simulink model "Correccion_Sist_Fisico_MA"  (R2021a)
settings: Solver=VariableStepAuto  StartTime=0.0  StopTime=inf  RelTol=1e-3
values from neighbouring files (symbols this model uses):
  b_cx = 1*10^6    (= 1000000)    [parametros.m]
  b_cy = 1*10^7    (= 10000000)    [parametros.m]
  b_eq = (b_td+b_tm*(r_t^2))/r_td    (= 10803.6)    [parametros.m]
  b_eqh = 2*(b_hd+b_hm*(r_h^2))/r_hd    (= 23253.3333333)    [parametros.m]
  b_ha = b_eqh/r_h - n_h*w_posh*(J_eqh + 0.5*m_l_*r_hd)/r_h    [parametros.m]
  b_hb = 1*10^8    (= 100000000)    [parametros.m]
  b_hEb = 2.2*10^9    (= 2200000000)    [parametros.m]
  b_t = 90    [parametros.m]
  b_ta = n_t*w_post*(r_td*J_eqt/r_t) - r_td*b_eqt/r_t    [parametros.m]
  b_tb = 5*10^6    (= 5000000)    [parametros.m]
  b_tw = 3*10^3    (= 3000)    [parametros.m]
  b_wu = 150    [parametros.m]
  dt = 5e-3    (= 0.005)    [parametros.m]
  g = 9.80665    [parametros.m]
  H_c = 2.5    [parametros.m]
  J_eq = (J_td+J_tm_tb*(r_t^2))/r_td    (= 15000)    [parametros.m]
  J_eqh = 2*(J_hd_hEb+J_hm_hb*(r_h^2))/r_hd    (= 48853.3333333)    [parametros.m]
  K_cy = 1.8*10^9    (= 1800000000)    [parametros.m]
  K_hsa = -n_h*(w_posh^2)*(J_eqh + 0.5*m_l_*r_hd)/r_t    [parametros.m]
  K_hsia = -(w_posh^3)*(J_eqh + 0.5*m_l_*r_hd)/r_t    [parametros.m]
  K_tsa = n_t*(w_post^2)*J_eqt*r_td/r_t    [parametros.m]
  K_tsia = (w_post^3)*J_eqt*r_td/r_t    [parametros.m]
  K_tw = 4.8*10^5    (= 480000)    [parametros.m]
  k_wu = 2.36*10^8    (= 236000000)    [parametros.m]
  lh_inicial = 45-yl_inicial    (= 30)    [parametros.m]
  M_c_MAX = 50000 + M_s    (= 65000)    [parametros.m]
  M_real = 10000    [parametros.m]
  M_s = 15000    [parametros.m]
  M_t = 30000    [parametros.m]
  r_h = 22    [parametros.m]
  r_hd = 0.75    [parametros.m]
  r_t = 30    [parametros.m]
  r_td = 0.5    [parametros.m]
  T_hb_MAX = 5*10^5    (= 500000)    [parametros.m]
  T_hEb_MAX = 1.1*10^6    (= 1100000)    [parametros.m]
  T_hm_MAX = 2*10^5    (= 200000)    [parametros.m]
  T_s2 = 5e-3    (= 0.005)    [parametros.m]
  T_tb_MAX = 5*10^4    (= 50000)    [parametros.m]
  T_tm_MAX = 3*10^4    (= 30000)    [parametros.m]
  tau_hm = 1e-3    (= 0.001)    [parametros.m]
  tau_tm = 1e-3    (= 0.001)    [parametros.m]
  TensionMinima = (M_s*g/2)*0.7    (= 51484.9125)    [parametros.m]
  v_h_MAX_c = +1.5    (= 1.5)    [parametros.m]
  v_t_MAX = +4    (= 4)    [parametros.m]
  v_t_MIN = -4    [parametros.m]
  w_hm_min = pi/4    (= 0.785398163397)    [parametros.m]
  w_tm_min = pi/4    (= 0.785398163397)    [parametros.m]
  xt_inicial = -10    [parametros.m]
  Y_t0 = 45    [parametros.m]
  yl_inicial = 15    [parametros.m]
undefined symbols (not defined in the file or in its folder): DiscIntNeverNeededParam
libraries: simulink x10, dspstat3 x1, vrlib x1
(part 3 of 3)

== stateflow chart Correccion_Sist_Fisico_MA/Chart ==
  note: ---> FINES DE CARRERA:
      |
      | 1. FIN DE CARRERA CARRO:
  state Nivel_1_Apagado
  note: ---> Si el Nivel 1 se encuentra apagodo deberia actuar el Nivel 0
  note: ---> Activado = Freno Energizado = Freno ABIERTO
  note: ---> Desactivado = Freno NO Energizado = Freno CERRADO
  state Nivel_1_Encendido
    state Sobrevelocidad [parallel]
      settings: executionOrder=11
      state CARRO [parallel]
        settings: executionOrder=2
        state Actualizacion_Vel_CARRO
          during:
          dx_t_SobreV = dx_t_ref_man;
        state Analisis_Sobrevelocidad
          entry:
          if (dx_t_ref_man>0)
          dx_t_SobreV = v_t_MAX;
          else
          dx_t_SobreV = v_t_MIN;
          end
        (default) -> Actualizacion_Vel_CARRO
        Actualizacion_Vel_CARRO -> Analisis_Sobrevelocidad : [abs(dx_t_ref_man) > v_t_MAX]
        Analisis_Sobrevelocidad -> Actualizacion_Vel_CARRO : [abs(dx_t_ref_man) <= v_t_MAX]
      state IZAJE [parallel]
        settings: executionOrder=1
        state Actualizacion_Vel_IZAJE
          during:
          dl_h_SobreV = dl_h_ref_man;
        state Analisis_Sobrevelocidad_Pos
          entry:
          dl_h_SobreV = v_h_MAXMIN;
        state Analisis_Sobrevelocidad_Neg
          entry:
          dl_h_SobreV = -v_h_MAXMIN;
        state BAJAR
          entry:
          dl_h_SobreV = v_h_MAX_c*0.1;
        (default) -> Actualizacion_Vel_IZAJE
        Actualizacion_Vel_IZAJE -> Analisis_Sobrevelocidad_Pos [order 1] : [(dl_h_ref_man > v_h_MAXMIN)  && ~sobrecarga ]
        Analisis_Sobrevelocidad_Pos -> Actualizacion_Vel_IZAJE : [(dl_h_ref_man <= v_h_MAXMIN) || sobrecarga ]
        Actualizacion_Vel_IZAJE -> Analisis_Sobrevelocidad_Neg [order 3] : [(dl_h_ref_man < -v_h_MAXMIN)   && ~sobrecarga ]
        Analisis_Sobrevelocidad_Neg -> Actualizacion_Vel_IZAJE : [(dl_h_ref_man >= -v_h_MAXMIN)  || sobrecarga ]
        Actualizacion_Vel_IZAJE -> BAJAR [order 2] : [sobrecarga]
        BAJAR -> Actualizacion_Vel_IZAJE : [~sobrecarga]
    state Fines_de_Carrera [parallel]
      settings: executionOrder=2
      state FIN_DE_CARRERA_CARRO [parallel]
        settings: executionOrder=1
        state Frenar
          entry:
          Detener_CarroFDC = 1;
        state MOVER_CARRO
          during:
          Detener_CarroFDC = 0;
        state No_Frenar
          entry:
          Detener_CarroFDC = 0;
        (default) -> Nivel_1_Encendido.Fines_de_Carrera.FIN_DE_CARRERA_CARRO.No_Frenar
        Nivel_1_Encendido.Fines_de_Carrera.FIN_DE_CARRERA_CARRO.Frenar -> Nivel_1_Encendido.Fines_de_Carrera.FIN_DE_CARRERA_CARRO.MOVER_CARRO [order 2] : [((dx_t_ref_man < 0 && Fin_Der_n) || (dx_t_ref_man > 0 && Fin_Izq_n))]
        Nivel_1_Encendido.Fines_de_Carrera.FIN_DE_CARRERA_CARRO.No_Frenar -> Nivel_1_Encendido.Fines_de_Carrera.FIN_DE_CARRERA_CARRO.Frenar : [Fin_Der_n || Fin_Izq_n]
        Nivel_1_Encendido.Fines_de_Carrera.FIN_DE_CARRERA_CARRO.MOVER_CARRO -> Nivel_1_Encendido.Fines_de_Carrera.FIN_DE_CARRERA_CARRO.Frenar : [(dx_t_ref_man >= 0 && Fin_Der_n) || (dx_t_ref_man <= 0 && Fin_Izq_n) || (~Fin_Der_n && ~Fin_Izq_n) ]
        Nivel_1_Encendido.Fines_de_Carrera.FIN_DE_CARRERA_CARRO.Frenar -> Nivel_1_Encendido.Fines_de_Carrera.FIN_DE_CARRERA_CARRO.No_Frenar [order 1] : [~Fin_Der_n && ~Fin_Izq_n]
      state FIN_DE_CARRERA_IZAJE [parallel]
        settings: executionOrder=2
        state Frenar
          entry:
          Detener_IzajeFDC = 1;
        state MOVER_IZAJE
          during:
          Detener_IzajeFDC = 0;
        state No_Frenar
          entry:
          Detener_IzajeFDC = 0;
        (default) -> Nivel_1_Encendido.Fines_de_Carrera.FIN_DE_CARRERA_IZAJE.No_Frenar
        Nivel_1_Encendido.Fines_de_Carrera.FIN_DE_CARRERA_IZAJE.Frenar -> Nivel_1_Encendido.Fines_de_Carrera.FIN_DE_CARRERA_IZAJE.MOVER_IZAJE [order 2] : [((dl_h_ref_man > 0 && Fin_Sup_n) || (dl_h_ref_man < 0 && Fin_Inf_n))]
        Nivel_1_Encendido.Fines_de_Carrera.FIN_DE_CARRERA_IZAJE.No_Frenar -> Nivel_1_Encendido.Fines_de_Carrera.FIN_DE_CARRERA_IZAJE.Frenar : [Fin_Sup_n || Fin_Inf_n]
        Nivel_1_Encendido.Fines_de_Carrera.FIN_DE_CARRERA_IZAJE.MOVER_IZAJE -> Nivel_1_Encendido.Fines_de_Carrera.FIN_DE_CARRERA_IZAJE.Frenar : [(dl_h_ref_man <= 0 && Fin_Sup_n) || (dl_h_ref_man >= 0 && Fin_Inf_n) || (~Fin_Sup_n && ~Fin_Inf_n) ]
        Nivel_1_Encendido.Fines_de_Carrera.FIN_DE_CARRERA_IZAJE.Frenar -> Nivel_1_Encendido.Fines_de_Carrera.FIN_DE_CARRERA_IZAJE.No_Frenar [order 1] : [~Fin_Sup_n && ~Fin_Inf_n]
    state Frenos [parallel]
      settings: executionOrder=4
      note: % Freno desactivado = Frenando
      state FRENO_CARRO [parallel]
        settings: executionOrder=1
        state No_Frenando
          entry:
          BRK_t = 1;
          Detener_CarroFR = 0;
        state Frenando
          entry:
          BRK_t = 0;
          Detener_CarroFR = 1;
        (default) -> Nivel_1_Encendido.Frenos.FRENO_CARRO.Frenando
        Nivel_1_Encendido.Frenos.FRENO_CARRO.No_Frenando -> Nivel_1_Encendido.Frenos.FRENO_CARRO.Frenando : [(abs(w_tm) < w_tm_min && Freno_Carro_Man) || (Emergencia == 2 && ~Salida_E_C) || sobrecarga || ( dx_t_ref == 0 && dx_t_SobreV == 0) ||  Detener_CarroFDC || (dx_t_ref * dx_t_ref_man < 0) ]
        Nivel_1_Encendido.Frenos.FRENO_CARRO.Frenando -> Nivel_1_Encendido.Frenos.FRENO_CARRO.No_Frenando : [Tmt_disp && ~Freno_Carro_Man && (Emergencia == 0 || Salida_E_C) && ~sobrecarga && ( dx_t_ref ~= 0 || dx_t_SobreV ~= 0) && ~Detener_CarroFDC && (dx_t_ref * dx_t_ref_man >= 0)]
      state FRENO_IZAJE [parallel]
        settings: executionOrder=2
        state No_Frenando
          entry:
          BRK_h = 1;
          Detener_IzajeFR = 0;
        state Frenando
          entry:
          BRK_h = 0;
          Detener_IzajeFR = 1;
        (default) -> Nivel_1_Encendido.Frenos.FRENO_IZAJE.Frenando
        Nivel_1_Encendido.Frenos.FRENO_IZAJE.No_Frenando -> Nivel_1_Encendido.Frenos.FRENO_IZAJE.Frenando : [(abs(w_hm) < w_hm_min && Freno_Izaje_Man) || (Emergencia == 3 && ~Salida_E_I)  || (sobrecarga && dl_h_ref <= 0) || ( dl_h_ref == 0 && dl_h_SobreV == 0) || Detener_IzajeFDC || ~Cable_Tenso || (45-l_h < y_obstaculo-0.15 && dl_h_ref_man >= 0) || (dl_h_ref * dl_h_ref_man < 0)]
        Nivel_1_Encendido.Frenos.FRENO_IZAJE.Frenando -> Nivel_1_Encendido.Frenos.FRENO_IZAJE.No_Frenando : [Tmh_disp && ~Freno_Izaje_Man && (Emergencia == 0 || Salida_E_I) && (~sobrecarga || sobrecarga && dl_h_ref > 0) && ( dl_h_ref ~= 0 || dl_h_SobreV ~= 0) && ~Detener_IzajeFDC && Cable_Tenso && (45-l_h >= y_obstaculo-0.15 || dl_h_ref_man < 0) && (dl_h_ref * dl_h_ref_man >= 0)]
      state FRENO_EMERGENCIA [parallel]
        settings: executionOrder=3
        state No_Frenando
          entry:
          BRK_hE = 1;
        state Frenando
          entry:
          BRK_hE = 0;
        (default) -> Nivel_1_Encendido.Frenos.FRENO_EMERGENCIA.Frenando
        Nivel_1_Encendido.Frenos.FRENO_EMERGENCIA.No_Frenando -> Nivel_1_Encendido.Frenos.FRENO_EMERGENCIA.Frenando : [~Grua_Encendida || (45-l_h < y_obstaculo-0.2 && dl_h_ref_man >= 0)]
        Nivel_1_Encendido.Frenos.FRENO_EMERGENCIA.Frenando -> Nivel_1_Encendido.Frenos.FRENO_EMERGENCIA.No_Frenando : [Grua_Encendida && (45-l_h > y_obstaculo-0.2 || dl_h_ref_man < 0)]
    state Sobrecarga [parallel]
      settings: executionOrder=7
      note: SI HAY SOBRECARGA SOLO SE PUEDE BAJAR MANUALMENTE
      state CON_SOBRECARGA
        entry:
        sobrecarga = 1;
      state SIN_SOBRECARGA
        entry:
        sobrecarga = 0;
      (default) -> SIN_SOBRECARGA
      SIN_SOBRECARGA -> CON_SOBRECARGA : [M_cX > M_c_MAX && MasaFija && TLK]
      CON_SOBRECARGA -> SIN_SOBRECARGA : [M_cX < M_c_MAX && MasaFija && ~TLK]
    state Twistlocks [parallel]
      settings: executionOrder=3
      note: SE ACTIVA EL TLK SI EL OPERARIO LO DESEA Y
          | ADEMAS LA TENSION EN EL CABLE ES 0 (spreader apoyado)
      state TLK_ABIERTO
        entry:
        TLK = 0;
        y_obstaculo = 0;
        during:
        y_obstaculo = Y_co;
      state TLK_CERRADO
        entry:
        TLK = 1;
        during:
        y_obstaculo = Y_co + 2.5;
      (default) -> TLK_ABIERTO
      TLK_CERRADO -> TLK_ABIERTO : [~Activar_TLK && ~Cable_Tenso && TLK]
      TLK_ABIERTO -> TLK_CERRADO : [Activar_TLK && ~Cable_Tenso && ~TLK]
    state Senal_Vida [parallel]
      settings: executionOrder=8
      state Pulso_alto
        entry:
        Vida=1;
      state Pulso_bajo
        entry:
        Vida=0;
      (default) -> Pulso_bajo
      Pulso_bajo -> Pulso_alto : after(500,msec)
      Pulso_alto -> Pulso_bajo : after(10,msec)
    state Deteccion_Cable_Flojo [parallel]
      settings: executionOrder=5
      state CABLE_TENSO
        entry:
        Cable_Tenso = 1;
      state CABLE_FLOJO
        entry:
        Cable_Tenso = 0;
      (default) -> CABLE_TENSO
      CABLE_FLOJO -> CABLE_TENSO : [dl_h_ref_man < 0 || F_hw > TensionMinima ]
      CABLE_TENSO -> CABLE_FLOJO : [dl_h_ref_man >= 0 && F_hw <= TensionMinima]
    state MOVER_GRUA_ESTADO_EMERGENCIA_CARRO [parallel]
      settings: executionOrder=10
      state MOVER_CARRO
        entry:
        Salida_E_C = 1;
      state INICIO
        entry:
        Salida_E_C = 0;
      state ESPERA
        Salida_E_C = 0;
      (default) -> INICIO
      ESPERA -> Nivel_1_Encendido.MOVER_GRUA_ESTADO_EMERGENCIA_CARRO.MOVER_CARRO [order 2] : [(dx_t_ref_man < 0 && Fin_Der_u) || (dx_t_ref_man > 0 && Fin_Izq_u)]
      INICIO -> ESPERA : [Emergencia == 2]
      Nivel_1_Encendido.MOVER_GRUA_ESTADO_EMERGENCIA_CARRO.MOVER_CARRO -> ESPERA : [(dx_t_ref_man >= 0 && Fin_Der_u) || (dx_t_ref_man <= 0 && Fin_Izq_u) || Emergencia == 0]
      ESPERA -> INICIO [order 1] : [Emergencia == 0]
    state Control_De_Balanceo [parallel]
      settings: executionOrder=6
      state ACTIVADO
        entry:
        BAC = 1;
      state DESACTIVADO
        entry:
        BAC = 0;
      (default) -> DESACTIVADO
      ACTIVADO -> DESACTIVADO : [~Balanceo || Emergencia ~=0]
      DESACTIVADO -> ACTIVADO : [Balanceo && Emergencia == 0]
    state MOVER_GRUA_ESTADO_EMERGENCIA_IZAJE [parallel]
      settings: executionOrder=9
      state MOVER_IZAJE
        entry:
        Salida_E_I = 1;
      state EMERGENCIA_IZAJE
        entry:
        Salida_E_I = 0;
      state NORMAL
        entry:
        Salida_E_I = 0;
      (default) -> NORMAL
      EMERGENCIA_IZAJE -> Nivel_1_Encendido.MOVER_GRUA_ESTADO_EMERGENCIA_IZAJE.MOVER_IZAJE [order 2] : [(dl_h_ref_man > 0 && Fin_Sup_u) || (dl_h_ref_man < 0 && Fin_Inf_u)]
      NORMAL -> EMERGENCIA_IZAJE : [Emergencia == 3]
      EMERGENCIA_IZAJE -> NORMAL [order 1] : [Emergencia == 0]
      Nivel_1_Encendido.MOVER_GRUA_ESTADO_EMERGENCIA_IZAJE.MOVER_IZAJE -> EMERGENCIA_IZAJE : [(dl_h_ref_man <= 0 && Fin_Sup_u) || (dl_h_ref_man >= 0 && Fin_Inf_u) || Emergencia == 0]
    state MODO [parallel]
      settings: executionOrder=12
      state MANUAL
        entry:
        Modo_Manual = 1;
        state Carro [parallel]
          settings: executionOrder=1
          state Operacion_Normal
            during:
            dx_t_ref = calcular_velocidad_maximaC(dx_t_SobreV);
          state sobrecarga_Carro
            entry:
            dx_t_ref = 0;
            calcular_velocidad_maximaC(0);
          state Analisis_FDC_D
            during:
            dx_t_ref = calcular_velocidad_maximaC(dx_t_SobreV*(50-x_td)/10);
          state Analisis_FDC_I
            during:
            dx_t_ref = calcular_velocidad_maximaC(dx_t_SobreV*(30+x_td)/10);
          state detener_carro
            entry:
            dx_t_ref = 0;
            calcular_velocidad_maximaC(0);
          (default) -> Nivel_1_Encendido.MODO.MANUAL.Carro.Operacion_Normal
          Analisis_FDC_D -> Nivel_1_Encendido.MODO.MANUAL.Carro.Operacion_Normal : [Detener_CarroFR || Detener_CarroFDC || dx_t_ref_man < 0]
          Nivel_1_Encendido.MODO.MANUAL.Carro.Operacion_Normal -> sobrecarga_Carro [order 1] : [sobrecarga]
          sobrecarga_Carro -> Nivel_1_Encendido.MODO.MANUAL.Carro.Operacion_Normal : [~sobrecarga]
          Nivel_1_Encendido.MODO.MANUAL.Carro.Operacion_Normal -> Analisis_FDC_D [order 3] : [x_td >=40 && dx_t_ref_man > 0 && ~Detener_CarroFR && ~Detener_CarroFDC && ~Fin_Der_n && ~Fin_Izq_n]
          Analisis_FDC_I -> Nivel_1_Encendido.MODO.MANUAL.Carro.Operacion_Normal : [Detener_CarroFR || Detener_CarroFDC || dx_t_ref_man > 0]
          Nivel_1_Encendido.MODO.MANUAL.Carro.Operacion_Normal -> detener_carro [order 2] : [Detener_CarroFR || Detener_CarroFDC ]
          Nivel_1_Encendido.MODO.MANUAL.Carro.Operacion_Normal -> Analisis_FDC_I [order 4] : [x_td <=-20 && dx_t_ref_man < 0 && ~Detener_CarroFR && ~Detener_CarroFDC]
          detener_carro -> Nivel_1_Encendido.MODO.MANUAL.Carro.Operacion_Normal : [~Detener_CarroFR  && ~Detener_CarroFDC ]
        state Izaje [parallel]
          settings: executionOrder=2
          note: dl_h_ref_man se refiere a longitud del cable. Si es >0, se tiene mayor longitud de cable y la carga baja. Si es <0 la longitud disminuye y la carga baja. El 5 en FDC_ARRIBA es una medida de seguridad. En estimacion de masa se limita la velocidad al 10%.
          state Operacion_Normal
            during:
            dl_h_ref = calcular_velocidad_maxima_I(dl_h_SobreV, MasaFija);
          state sobrecarga_Izaje
            during:
            if (dl_h_ref_man>0)
            dl_h_ref = calcular_velocidad_maxima_I(dl_h_SobreV, MasaFija);
            else
            dl_h_ref = 0;
            calcular_velocidad_maxima_I(0, MasaFija);
            end
          state Analisis_FDC_ARRIBA
            during:
            dl_h_ref = calcular_velocidad_maxima_I(dl_h_SobreV*(l_h-5)/5, MasaFija);
          state Analisis_FDC_ABAJO
            during:
            dl_h_ref = calcular_velocidad_maxima_I(dl_h_SobreV*(65-l_h)/10, MasaFija);
          state detener_Izaje
            entry:
            dl_h_ref = 0;
            calcular_velocidad_maxima_I(0, MasaFija);
          state Analisis_ESTIMACION_MASA
            during:
            dl_h_ref = calcular_velocidad_maxima_I(dl_h_SobreV, MasaFija)*0.1;
          state Analisis_OBSTACULO
            during:
            dl_h_ref = calcular_velocidad_maxima_I(dl_h_SobreV*(45-y_obstaculo-l_h+0.2)/5, MasaFija);
          (default) -> Nivel_1_Encendido.MODO.MANUAL.Izaje.Operacion_Normal
          Analisis_FDC_ARRIBA -> Nivel_1_Encendido.MODO.MANUAL.Izaje.Operacion_Normal : [Detener_IzajeFR || Detener_IzajeFDC || dl_h_ref_man > 0]
          Nivel_1_Encendido.MODO.MANUAL.Izaje.Operacion_Normal -> sobrecarga_Izaje [order 1] : [sobrecarga]
          Nivel_1_Encendido.MODO.MANUAL.Izaje.Operacion_Normal -> Analisis_FDC_ARRIBA [order 4] : [l_h <=10 && dl_h_ref_man < 0 && ~Detener_IzajeFR && ~Detener_IzajeFDC]
          sobrecarga_Izaje -> Nivel_1_Encendido.MODO.MANUAL.Izaje.Operacion_Normal : [~sobrecarga]
          Analisis_FDC_ABAJO -> Nivel_1_Encendido.MODO.MANUAL.Izaje.Operacion_Normal : [Detener_IzajeFR || Detener_IzajeFDC  || dl_h_ref_man < 0]
          Nivel_1_Encendido.MODO.MANUAL.Izaje.Operacion_Normal -> Analisis_FDC_ABAJO [order 5] : [l_h >=55 && dl_h_ref_man > 0 && ~Detener_IzajeFR && ~Detener_IzajeFDC]
          Analisis_ESTIMACION_MASA -> Nivel_1_Encendido.MODO.MANUAL.Izaje.Operacion_Normal : [MasaFija || sobrecarga || Detener_IzajeFR || Detener_IzajeFDC]
          Nivel_1_Encendido.MODO.MANUAL.Izaje.Operacion_Normal -> detener_Izaje [order 2] : [(Detener_IzajeFR || Detener_IzajeFDC) && ~sobrecarga]
          detener_Izaje -> Nivel_1_Encendido.MODO.MANUAL.Izaje.Operacion_Normal : [(~Detener_IzajeFR && ~Detener_IzajeFDC) || sobrecarga]
          Nivel_1_Encendido.MODO.MANUAL.Izaje.Operacion_Normal -> Analisis_ESTIMACION_MASA [order 6] : [~MasaFija && TLK && ~Detener_IzajeFR && ~Detener_IzajeFDC && Cable_Tenso]
          Analisis_OBSTACULO -> Nivel_1_Encendido.MODO.MANUAL.Izaje.Operacion_Normal : [Detener_IzajeFR || Detener_IzajeFDC  || dl_h_ref_man < 0]
          Nivel_1_Encendido.MODO.MANUAL.Izaje.Operacion_Normal -> Analisis_OBSTACULO [order 3] : [(y_obstaculo+5) >= (45-l_h) && dl_h_ref_man > 0 && ~Detener_IzajeFR && ~Detener_IzajeFDC]
      state AUTOMATICO
        entry:
        esperando_estabilizacion=true;
        punto_lim = [0, 10];
        punto_muelle = [-20, 4.5];
        during:
        if MasaFija && esperando_estabilizacion
        y_l = pos_y_actual(l_h, TLK);
        punto_in = [x_td, y_l];
        %if TLK && Cable_Tenso
        %    [trayectoria_x, trayectoria_y] = generar_trayectoria_vuelta(y_max, punto_lim, punto_in, punto_muelle);
        %else
        %   posicion_final = obtener_pos_final(contenedor_posiciones)
        %  [trayectoria_x, trayectoria_y] = generar_trayectoria_ida(y_max, punto_lim, punto_in, posicion_final);
        %end
        [perfil_velocidad_x, perfil_velocidad_y, cant_x, cant_y] = obtener_perfil_velocidad([-10, 10, 15], [15, 20, 20], TLK);
        it_x = 1;
        it_y = 1;
        esperando_estabilizacion = false;
        end
        if ~esperando_estabilizacion
        if it_x <= cant_x
        dx_t_ref = perfil_velocidad_x(it_x, 2);
        else
        dx_t_ref = 0;
        end
        if it_y <= cant_y
        dl_h_ref = -perfil_velocidad_y(it_y, 2);
        else
        dl_h_ref = 0;
        end
        it_x = it_x + 1;
        it_y = it_y + 1;
        end
      (default) -> MANUAL
      MANUAL -> AUTOMATICO : [Cambiar_Modo && ~IteracionTerminada]
      AUTOMATICO -> MANUAL : [~Cambiar_Modo || IteracionTerminada]
    state OBSTACULOS [parallel]
      entry:
      [contenedor_posiciones, y_max] = actualizar_contenedores(contenedor_pos_iniciales, -10, 10); % Pongo valor random para q me devuelva
      matriz_Y_co = calculo_matriz_yc0(contenedor_posiciones)                                                        % el y_max y no hacer otra funcion
      settings: executionOrder=1
      state ACTUALIZACION_CONTENEDORES [parallel]
        settings: executionOrder=1
        state Verificar
        state Carga
          entry:
          y_actual = pos_y_actual(l_h, TLK);
          [contenedor_posiciones, y_max] = actualizar_contenedores(contenedor_posiciones, x_td, y_actual);
          matriz_Y_co = calculo_matriz_yc0(contenedor_posiciones);
        state Descarga
          entry:
          % Por ahora no hace nada, va a servir para los otros modos
        (default) -> Verificar
        Verificar -> Carga [order 1] : [~Cable_Tenso &&  Activar_TLK && ~TLK ]
        Carga -> Verificar : [Cable_Tenso && MasaFija]
        Verificar -> Descarga [order 2] : [Cable_Tenso &&  ~Activar_TLK && TLK ]
        Descarga -> Verificar : [~Cable_Tenso]
      state CALCULAR_YCO [parallel]
        settings: executionOrder=2
        state Calculo_YC0
          during:
          Y_co = obtener_Y_c0(matriz_Y_co, x_td);
        (default) -> Calculo_YC0
  (default) -> Nivel_1_Apagado
  Nivel_1_Apagado -> Nivel_1_Encendido : [Alimentacion]
  Nivel_1_Encendido -> Nivel_1_Apagado : [~Alimentacion]
  data: dx_manual function_input; v_max_carro function_output; dh_manual function_input; v_max_izaje function_output; Enclave function_input; contenedor_pos function_output; contenedor_pos function_input; pos_x function_input; pos_y function_input; y_superior function_output; y_superior function_input; p_lim function_input; p_inicial function_input; punto_final function_input; tray_x function_output; tray_y function_output; matriz_yc0 function_output; contenedor_pos function_input; contenedor_pos function_input; p_final function_output; matriz_yc0 function_input; yc0 function_output; xtd function_input; y_superior function_input; p_lim function_input; p_inicial function_input; punto_final function_input; tray_x function_output; tray_y function_output; l function_input; tlk function_input; pos_y function_output; puntos_x function_input; puntos_y function_input; cargado function_input; perfil_vel_x function_output; perfil_vel_y function_output; cantidad_puntos_x function_output; cantidad_puntos_y function_output; Alimentacion input; Fin_Der_n input; Fin_Izq_n input; Fin_Sup_n input; Fin_Inf_n input; BRK_t output; BRK_h output; BRK_hE output; Vida output size=1; Emergencia input; Grua_Encendida input; dx_t_ref_man input; dl_h_ref_man input; w_tm input; w_hm input; Freno_Carro_Man input; Freno_Izaje_Man input; Balanceo input; x_td input; l_h input; MasaFija input; Activar_TLK input; M_cX input; dx_t_ref output =0; dl_h_ref output =0; BAC output; TLK output size=1; v_t_MAX parameter; v_t_MIN parameter; Tmt_disp input; w_tm_min parameter; w_hm_min parameter; Tmh_disp input; F_hw input; v_h_MAX_c parameter; Modo_Manual output size=1; Cable_Tenso local; dx_t_SobreV local =0; dl_h_SobreV local =0; sobrecarga local; M_c_MAX parameter; TensionMinima parameter; v_h_MAXMIN input; Detener_IzajeFDC local; Detener_CarroFDC local; Detener_CarroFR local; Detener_IzajeFR local; Fin_Sup_u input; Fin_Inf_u input; Fin_Izq_u input; Fin_Der_u input; Salida_E_C local; Salida_E_I local; y_obstaculo local; esperando_estabilizacion local; punto_muelle local; posicion_final local size=1,2 =0,0; y_l local; posicion_y_actual local size=1 =yl_inicial; y_max local; y_actual local; matriz_Y_co local size=1,16; contenedor_posiciones local size=18,16; contenedor_pos_iniciales input; Y_co output size=1; punto_in local; punto_lim local; trayectoria_x local size=[1,10]; trayectoria_y local size=[1,10]; cant_puntos_discretizacion local size=1 =0; it local size=1 =0; perfil_velocidad_y local double size=100000,2; perfil_velocidad_x local double size=100000,2; Cambiar_Modo input; IteracionTerminada local size=1 =false; cant_y local double size=1; it_x local double size=1; it_y local double size=1; cant_x local double size=1
  function v_max_carro = calcular_velocidad_maximaC(dx_manual):
    | function v_max_carro = calcular_velocidad_maximaC(dx_manual)
    | 
    | %--------------------------------------------------------------------------%
    | %---------------------Declaracion variables PERSISTENT---------------------% 
    | %--------------------------------------------------------------------------%
    |             % --> Persistent: local variable in a function that retains its 
    |                             % value in memory between calls to the function
    |     persistent dx_t_ref_manual_anterior;
    |     a_max_carro = 1;     % m/s^2 (aceleracion max para el subsistema carro)
    |     dt = 0.02;           % 20 ms (tiempo de muestreo del statechart)
    |     
    | %--------------------------------------------------------------------------%
    | %------------------Inicialización de variables PERSISTENT------------------% 
    | %--------------------------------------------------------------------------%
    | 
    |     if isempty(dx_t_ref_manual_anterior)
    |         dx_t_ref_manual_anterior = 0;
    |     end
    |     
    | %--------------------------------------------------------------------------%
    | %-----------------------------Lógica principal-----------------------------%
    | %--------------------------------------------------------------------------%
    | % La idea es que el sistema siempre vaya a la maxima velocidad que pueda.
    | % Para eso se utiliza la aceleracion maxima para el subsistema carro en
    | % caso de que la velocidad de referencia no sea lo suficientemente grande.
    | % Si la velocidad supera la velocidad maxima, esta se limita al maximo
    | % permitido.
    |     if (dx_manual == 0)
    |         v_max_carro_aux = 0;
    |     else
    |         if abs(dx_manual) >= abs(dx_t_ref_manual_anterior)
    |             if dx_manual > 0                                                    % Aceleracion +
    |                 v_max = a_max_carro * dt + dx_t_ref_manual_anterior;
    |                 v_max_carro_aux = max(v_max, dx_manual);
    |             else                                                                % Aceleracion -
    |                 v_max = -a_max_carro * dt + dx_t_ref_manual_anterior;
    |                 v_max_carro_aux = min(v_max, dx_manual);
    |             end
    |         elseif dx_manual < dx_t_ref_manual_anterior                             % Desaceleracion -
    |             v_max = -a_max_carro * dt + dx_t_ref_manual_anterior;
    |             v_max_carro_aux = min(v_max, dx_manual);
    |         else                                                                    % Desaceleracion +
    |             v_max = a_max_carro * dt + dx_t_ref_manual_anterior;
    |             v_max_carro_aux = max(v_max, dx_manual);
    |         end
    | 
    |         if abs(v_max_carro_aux) > 4
    |             if v_max_carro_aux > 0
    |                 v_max_carro_aux = 4;
    |             else
    |                 v_max_carro_aux = -4;
    |             end
    |         end
    |     end
    |     v_max_carro = v_max_carro_aux;
    | 
    |     dx_t_ref_manual_anterior = v_max_carro;
    | end
  function v_max_izaje =   calcular_velocidad_maxima_I(dh_manual, Enclave):
    | function v_max_izaje =   calcular_velocidad_maxima_I(dh_manual, Enclave) % CT es Cable Tenso
    | 
    | %--------------------------------------------------------------------------%
    | %---------------------Declaracion variables PERSISTENT---------------------% 
    | %--------------------------------------------------------------------------%
    |             % --> Persistent: local variable in a function that retains its 
    |                             % value in memory between calls to the function
    |     persistent dy_href_manual_ant;
    |     persistent a_max_y;  % m/s^2
    |     persistent dt;       % 20 ms (tiempo de muestreo del statechart)
    |     
    | %--------------------------------------------------------------------------%
    | %------------------Inicialización de variables PERSISTENT------------------% 
    | %--------------------------------------------------------------------------%
    | 
    |     if isempty(dy_href_manual_ant)
    |         dy_href_manual_ant = 0;
    |     end
    |     if isempty(a_max_y)
    |         a_max_y = 0.75;  % m/s^2
    |     end
    |     if isempty(dt)
    |         dt = 0.02;       % 20 ms (tiempo de muestreo del statechart)
    |     end
    |     
    | %--------------------------------------------------------------------------%
    | %-----------------------------Lógica principal-----------------------------%
    | %--------------------------------------------------------------------------%
    | % La idea es que el sistema siempre vaya a la maxima velocidad que pueda.
    | % Para eso se utiliza la aceleracion maxima para el subsistema carro en
    | % caso de que la velocidad de referencia no sea lo suficientemente grande.
    | % Si la velocidad supera la velocidad maxima, esta se limita al maximo
    | % permitido.
    |     if (dh_manual ==0)
    |         v_max_izaje_aux = 0;
    |     else
    |         if abs(dh_manual) >= abs(dy_href_manual_ant)
    |             if dh_manual > 0
    |                 v_max = a_max_y * dt + dy_href_manual_ant;
    |                 v_max_izaje_aux = max(v_max, dh_manual);
    |             else
    |                 v_max = -a_max_y * dt + dy_href_manual_ant;
    |                 v_max_izaje_aux = min(v_max, dh_manual);
    |             end
    |         else
    |             if dh_manual < dy_href_manual_ant
    |                 v_max = -a_max_y * dt + dy_href_manual_ant;
    |                 v_max_izaje_aux = min(v_max, dh_manual);
    |             else
    |                 v_max = a_max_y * dt + dy_href_manual_ant;
    |                 v_max_izaje_aux = max(v_max, dh_manual);
    |             end
    |         end
    | 
    |         if Enclave == 1      % Hay carga, velocidad maxima 1.5 m/s
    |             if abs(v_max_izaje_aux) > 1.5
    |                 if v_max_izaje_aux > 0
    |                     v_max_izaje_aux = 1.5;
    |                 else
    |                     v_max_izaje_aux = -1.5;
    |                 end
    |             end
    |         else                % No hay carga, velocidad maxima 3 m/s
    |             if abs(v_max_izaje_aux) > 3
    |                 if v_max_izaje_aux > 0
    |                     v_max_izaje_aux = 3;
    |                 else
    |                     v_max_izaje_aux = -3;
    |                 end
    |             end
    |         end
    |     end
    |     v_max_izaje = v_max_izaje_aux;
    |     dy_href_manual_ant = v_max_izaje;
    | 
    | end
  function [contenedor_pos, y_superior] = actualizar_contenedores(contenedor_pos, pos_x, pos_y):
    | function [contenedor_pos, y_superior] = actualizar_contenedores(contenedor_pos, pos_x, pos_y)
    |     for columna = 1:size(contenedor_pos, 2)
    |         cantidad_contenedores_columna = sum(contenedor_pos(:,columna));
    |         if cantidad_contenedores_columna ~= 0 % Es decir si quedan contenedores en esa columna
    |             pos_x_izq_contenedor = 2.5 + (columna - 1) * 3;
    |             pos_x_der_contenedor = pos_x_izq_contenedor + 2.5;
    |             tolerancia = 0.2;
    |             pos_y_superior_contenedor = cantidad_contenedores_columna * 2.5 + tolerancia;
    |             if pos_x > pos_x_izq_contenedor && pos_x < pos_x_der_contenedor && pos_y < pos_y_superior_contenedor 
    |                 contenedor_pos(cantidad_contenedores_columna, columna) = 0;
    |                 break;
    |             end
    |         end
    |     end
    |     unos_por_columna = sum(contenedor_pos); % Me da la suma de cada columna
    |     max_contenedores = max(unos_por_columna); % Busco el máximo de la suma de cada columna
    |     
    |     coef_seguridad = 5;
    |     y_superior = max_contenedores*2.5 + coef_seguridad;
    | end
  function [tray_x, tray_y] = generar_trayectoria_vuelta(y_superior, p_lim, p_inicial, punto_final):
    | function [tray_x, tray_y] = generar_trayectoria_vuelta(y_superior, p_lim, p_inicial, punto_final)
    |     % Parámetros
    |     grados = 30;
    |     coef_seguridad = 3;
    |     altura_bajar = 25; % Altura desde donde empieza a bajar en línea recta
    | 
    |     % Ajustes iniciales
    |     p_lim(2) = p_lim(2) + coef_seguridad;
    |     tang = tan(grados*pi/180);
    | 
    |     % Inicializar trayectoria
    |     tray_x = p_inicial(1);
    |     tray_y = p_inicial(2);
    |     pos_actual = p_inicial;
    | 
    |     % Primer y segundo tramo (subir en línea recta y subir en oblicuo)
    |     puede_subir = false;
    |     dist = tang * (y_superior - pos_actual(2));
    |     while ~puede_subir
    |         dist = tang * (y_superior - pos_actual(2));
    |         m = (y_superior - pos_actual(2)) / ((pos_actual(1) - dist) - pos_actual(1));
    |         b = pos_actual(2) - m * pos_actual(1);
    | 
    |         interseccion_x = m * p_lim(1) + b;
    |         interseccion_y = (p_lim(2) - b) / m;
    | 
    |         if interseccion_x <= p_lim(2) || interseccion_x <= p_lim(1)
    |             pos_actual = [pos_actual(1), pos_actual(2) + 0.5];
    |             tray_x = [tray_x, pos_actual(1)];
    |             tray_y = [tray_y, pos_actual(2)];
    |         else
    |             puede_subir = true;
    |         end
    |     end
    |     
    |     % Ajuste de posición después de subir en oblicuo
    |     pos_actual(1) = pos_actual(1) - dist;
    |     pos_actual(2) = y_superior;
    |     tray_x = [tray_x, pos_actual(1)];
    |     tray_y = [tray_y, pos_actual(2)];
    | 
    |     % Tercer tramo (línea recta horizontal)
    |     punto_final_linea_recta = [punto_final(1) + tang * (y_superior - altura_bajar), y_superior];
    |     if punto_final_linea_recta(1) < pos_actual(1)
    |         tray_x = [tray_x, punto_final_linea_recta(1)];
    |         tray_y = [tray_y, punto_final_linea_recta(2)];
    |     end
    | 
    |     % Cuarto tramo (bajar en oblicuo)
    |     tray_x = [tray_x, punto_final(1)];
    |     tray_y = [tray_y, punto_final(2) + altura_bajar];
    | 
    |     % Quinto tramo (bajar en línea recta)
    |     tray_x = [tray_x, punto_final(1)];
    |     tray_y = [tray_y, punto_final(2)];
    | end
  function matriz_yc0 = calculo_matriz_yc0(contenedor_pos):
    | function matriz_yc0 = calculo_matriz_yc0(contenedor_pos)
    |     cant_columnas = size(contenedor_pos, 2);
    |     matriz_yc0 = zeros(1,cant_columnas);
    |     for columna = 1:cant_columnas
    |         cantidad_contenedores_columna = sum(contenedor_pos(:,columna));
    |         matriz_yc0(1,columna) = cantidad_contenedores_columna * 2.5 - 20; % -20 es la posición donde arrancan los contenedores a apoyarse
    |     end
    | end
  function p_final = obtener_pos_final(contenedor_pos):
    | function p_final = obtener_pos_final(contenedor_pos)
    |     p_final = [0, 0];
    |     posicion_encontrada = false;
    |     % En principio busca posiciones de izquierda a derecha de los
    |     % contenedores
    |     for columna = 1:size(contenedor_pos, 2)
    |         cantidad_contenedores_columna = sum(contenedor_pos(:,columna));
    |         if cantidad_contenedores_columna ~= 0 % Es decir si quedan contenedores en esa columna
    |             altura_a_manual = 2.5;
    |             posicion_encontrada = true;
    |             p_final = [2.5 + (columna * 3 - 0.5)/2, cantidad_contenedores_columna * 2.5 + altura_a_manual];
    |             % 2.5 es donde inician los contenedores, 3 es la separación
    |             % entre el inicio de uno y inicio de otro, 0.5 es la
    |             % separación entre los dos y dos porque damos la posición
    |             % central en x
    |             break;
    |         end
    |     end
    |     if ~posicion_encontrada
    |         p_final = [-30, 40]; % Lo pongo en la esquina superior izquierda.
    |     end
    | end
  function yc0 = obtener_Y_c0(matriz_yc0, xtd):
    | function yc0 = obtener_Y_c0(matriz_yc0, xtd)
    |     yc0 = 0;
    |     if xtd >= 2.5 && xtd <= 48
    |         % 2.5 es donde empiezan los contenedores
    |         % 48 sería 3 (que es la distancia desde la parte izq del contenedor y la izq del siguiente)
    |         % por 16 columnas de contenedores
    |         coef_seguridad = 0.5;
    |         yc0 = matriz_yc0(1,ceil(xtd/3)) + coef_seguridad;
    |     end
    | end
  function [tray_x, tray_y] = generar_trayectoria_ida(y_superior, p_lim, p_inicial, punto_final):
    | function [tray_x, tray_y] = generar_trayectoria_ida(y_superior, p_lim, p_inicial, punto_final)
    |     % Parámetros
    |     grados = 30;
    |     coef_seguridad = 3;
    | 
    |     % Ajustes iniciales
    |     p_lim(2) = p_lim(2) + coef_seguridad;
    |     tang = tan(grados*pi/180);
    | 
    |     % Inicializar trayectoria
    |     tray_x = p_inicial(1);
    |     tray_y = p_inicial(2);
    |     pos_actual = p_inicial;
    | 
    |     % Verificar si está cerca del borde del muelle para subir directamente
    |     if pos_actual(1) < -5
    |         % Si la pos_actual es mayor a la y_superior directamente va a avanzar
    |         if pos_actual(2) < y_superior
    |             % Primer tramo (subir línea recta)
    |             altura_subir_bajar = 25;
    |             punto_a_subir = pos_actual(2) + altura_subir_bajar;
    | 
    |             % Verificar si puede hacer un primer tramo en línea recta sin superar la parte superior
    |             if punto_a_subir < y_superior
    |                 pos_actual(2) = punto_a_subir;
    |                 tray_x = [tray_x, pos_actual(1)];
    |                 tray_y = [tray_y, pos_actual(2)];
    |             end
    | 
    |             % Segundo tramo (subir oblicuo)
    |             pos_actual(1) = pos_actual(1) + tang * (y_superior - pos_actual(2));
    |             pos_actual(2) = y_superior;
    |             tray_x = [tray_x, pos_actual(1)];
    |             tray_y = [tray_y, pos_actual(2)];   
    |         end
    | 
    |     else
    |         % Primer tramo (subir/bajar línea recta)
    |         pos_actual(2) = y_superior;
    |         tray_x = [tray_x, pos_actual(1)];
    |         tray_y = [tray_y, pos_actual(2)];
    |     end
    | 
    |     % Tercer y cuarto tramo (avanzar en horizontal y bajar en oblicuo)
    |     puede_bajar = false;
    |     while ~puede_bajar
    |         m = (punto_final(2) - y_superior) / (punto_final(1) - pos_actual(1));
    |         b = pos_actual(2) - m * pos_actual(1);
    | 
    |         interseccion_x = m * p_lim(1) + b;
    |         interseccion_y = (p_lim(2) - b) / m;
    | 
    |         if interseccion_x <= p_lim(2) || interseccion_x <= p_lim(1)
    |             pos_actual = [pos_actual(1) + 0.5, pos_actual(2)];
    |             tray_x = [tray_x, pos_actual(1)];
    |             tray_y = [tray_y, pos_actual(2)];
    |         else
    |             puede_bajar = true;
    |         end
    |     end
    | 
    |     % Quinto tramo (bajar en línea recta)
    |     tray_x = [tray_x, punto_final(1)];
    |     tray_y = [tray_y, punto_final(2)];
    | end
  function pos_y = pos_y_actual(l, tlk):
    | function pos_y = pos_y_actual(l, tlk)
    |     if tlk
    |         pos_y=45-l-2.5;
    |     else
    |         pos_y=45-l;
    |     end
    | end
  function [perfil_vel_x, perfil_vel_y, cantidad_puntos_x, cantidad_puntos_y] = obtener_perfil_velocidad(puntos_x, puntos_y, cargado):
    | function [perfil_vel_x, perfil_vel_y, cantidad_puntos_x, cantidad_puntos_y] = obtener_perfil_velocidad(puntos_x, puntos_y, cargado)
    |     % Obtener parámetros de aceleración y velocidad máxima
    |     tipo = 'carro';
    |     [a_max, v_max] = obtenerParametros(tipo, cargado);
    |     perfil_vel_x = obtener_perfil_vel(puntos_x, puntos_y, a_max, v_max, tipo, cargado);
    |     
    |     tipo = 'izaje';
    |     [a_max, v_max] = obtenerParametros(tipo, cargado);
    |     perfil_vel_y = obtener_perfil_vel(puntos_y, puntos_x, a_max, v_max, tipo, cargado);
    | 
    |     tiempo_total_x = perfil_vel_x(end,1);
    |     tiempo_total_y = perfil_vel_y(end,1);
    |     
    |     cantidad_puntos_x = floor(tiempo_total_x / 5e-3);
    |     cantidad_puntos_y = floor(tiempo_total_y / 5e-3);
    | 
    |     
    |     % Discretizar el perfil de velocidad al final
    |     % La opción 'pchip' en interp1 realiza una interpolación cúbica
    |     
    |     t_vals_discretizados_x = linspace(perfil_vel_x(1, 1), perfil_vel_x(end, 1), cantidad_puntos_x);
    |     v_vals_discretizados_x = interp1(perfil_vel_x(:, 1), perfil_vel_x(:, 2), t_vals_discretizados_x, 'linear');
    |     
    |     t_vals_discretizados_y = linspace(perfil_vel_y(1, 1), perfil_vel_y(end, 1), cantidad_puntos_y);
    |     v_vals_discretizados_y = interp1(perfil_vel_y(:, 1), perfil_vel_y(:, 2), t_vals_discretizados_y, 'linear');
    |     
    |     perfil_vel_x = [t_vals_discretizados_x', v_vals_discretizados_x'];
    |     perfil_vel_y = [t_vals_discretizados_y', v_vals_discretizados_y'];
    | end
    | 
    | function [a_max, v_max] = obtenerParametros(tipo, cargado)
    |     switch tipo
    |         case 'carro'
    |             a_max = 1;
    |             v_max = 4;
    |         otherwise
    |             a_max = 0.75;
    |             v_max = cargado * 1.5 + ~cargado * 3;
    |     end
    | end
    | 
    | function perfil_vel = obtener_perfil_vel(puntos, puntos_aux, a_max, v_max, tipo, cargado)
    |     % Inicializar el perfil de velocidad
    |     perfil_vel = zeros(1, 2);
    |     
    |     % Calcular el tiempo de transición
    |     t_trans = v_max / a_max;
    |     
    |     % Iterar sobre los puntos
    |     t_ant = 0;
    |     for i = 1:numel(puntos)-1
    |         dist = puntos(i+1) - puntos(i);
    |         abs_dist = abs(dist);
    |         
    |         % Calcular tiempo en tramo constante
    |         t_cte = abs_dist / v_max - t_trans;
    |         
    |         if t_cte > 0
    |             % Tramo con velocidad constante
    |             perfil_vel = [perfil_vel; 
    |                 t_ant + t_trans, sign(dist)*v_max; 
    |                 t_ant + t_trans + t_cte, sign(dist)*v_max; 
    |                 t_ant + t_trans*2 + t_cte, 0];
    |         elseif t_cte == 0
    |             % Tramo sin velocidad constante pero llegando a la v_max
    |             perfil_vel = [perfil_vel; 
    |                 t_ant + t_trans, sign(dist)*v_max; 
    |                 t_ant + t_trans*2, 0];
    |         else
    |             if abs_dist ~= 0
    |                 % Tramo sin velocidad constante sin llegar a la v_max
    |                 v_x = sqrt(a_max*abs_dist);
    |                 t_x = abs_dist/v_x;
    |                 perfil_vel = [perfil_vel; 
    |                     t_ant + t_x, sign(dist)*v_x; 
    |                     t_ant + t_x*2, 0];
    |             else
    |                 % Básicamente acá tiene que esperar a que se mueva el otro
    |                 % eje
    |                 tiempo = obtener_tiempo_espera(i, puntos_aux, tipo, cargado)
    |                 perfil_vel = [perfil_vel; t_ant + tiempo, 0];
    |             end
    |         end
    |         
    |         % Actualizar tiempo anterior
    |         t_ant = perfil_vel(end, 1);
    |     end
    | end
    | 
    | function tiempo = obtener_tiempo_espera(i, puntos, tipo, cargado)
    |     if tipo == 'carro'
    |         tipo = 'izaje'
    |     else
    |         tipo = 'carro'
    |     end
    |     [a_max, v_max] = obtenerParametros(tipo, cargado);
    |     perfil_vel = zeros(1, 2);
    |     % Calcular el tiempo de transición
    |     t_trans = v_max / a_max;
    |     tiempo = 0;
    |     t_ant = 0;
    |     dist = puntos(i+1) - puntos(i);
    |     abs_dist = abs(dist);
    |     
    |     % Calcular el tiempo de transición
    |     t_trans = v_max / a_max;
    |     
    |     % Calcular tiempo en tramo constante
    |     t_cte = abs_dist / v_max - t_trans;
    | 
    |     if t_cte > 0
    |         % Tramo con velocidad constante
    |         perfil_vel = [perfil_vel; 
    |             t_ant + t_trans, sign(dist)*v_max; 
    |             t_ant + t_trans + t_cte, sign(dist)*v_max; 
    |             t_ant + t_trans*2 + t_cte, 0];
    |     elseif t_cte == 0
    |         % Tramo sin velocidad constante pero llegando a la v_max
    |         perfil_vel = [perfil_vel; 
    |             t_ant + t_trans, sign(dist)*v_max; 
    |             t_ant + t_trans*2, 0];
    |     else
    |         if abs_dist ~= 0
    |             % Tramo sin velocidad constante sin llegar a la v_max
    |             v_x = sqrt(a_max*abs_dist);
    |             t_x = abs_dist/v_x;
    |             perfil_vel = [perfil_vel; 
    |                 t_ant + t_x, sign(dist)*v_x; 
    |                 t_ant + t_x*2, 0];
    |         end
    |     end
    | 
    |     tiempo = perfil_vel(end,1);
    | end
